simulink model "foptdModel_21a"  (Simulink 10.3)
settings: Solver=FixedStepAuto  StartTime=0.0  StopTime=toutReal(end)-0.3  FixedStep=0.3  RelTol=1e-3
values from neighbouring files (symbols this model uses):
  deltap = [10.95 6 7.8 19.65 17.55 2.85 17.7]    [SimulinkFOPTD-DESKTOP-H1.m]    (also in SimulinkFOPTD.m)
  du = 0.5    [SimulinkFOPTD-DESKTOP-H1.m]    (also in SimulinkFOPTD.m)
  i = input("Wybierz numer skoku (1-7): ")    [SimulinkFOPTD-DESKTOP-H1.m]    (also in SimulinkFOPTD.m)
  taup = [60.75 42.3 39.6 41.85 39.15 20.25 30.6]    [SimulinkFOPTD-DESKTOP-H1.m]    (also in SimulinkFOPTD.m)
  y0 = [59.8 48.9 42.1 37.4 34 31.6 29.7]    [SimulinkFOPTD-DESKTOP-H1.m]    (also in SimulinkFOPTD.m)
undefined symbols (not defined in the file or in its folder): K
settings Model: Creator=danie  LastModifiedBy=hkacp
settings SolverCC: AlgebraicLoopSolver=Auto
settings DataIOCC: SaveFormat=Dataset  SignalLoggingSaveFormat=Dataset  ReturnWorkspaceOutputs=on
settings OptimizationCC: ExpressionDepthLimit=128  LifeSpan=auto
settings DebuggingCC: UnderspecifiedInitializationDetection=Simplified  MergeDetectMultiDrivingBlocksExec=error  FcnCallInpInsideContextMsg=error  StateNameClashWarn=none  SFUnexpectedBacktrackingDiag=error  SFNoUnconditionalDefaultTransitionDiag=error  SFExecutionAtInitializationDiag=warning  SFMachineParentedDataDiag=error  ArithmeticOperatorsInVariantConditions=error
settings HardwareCC: ProdBitPerPointer=64  ProdBitPerSizeT=64  ProdBitPerPtrDiffT=64  ProdLargestAtomicFloat=Float  ProdIntDivRoundTo=Zero  ProdEndianess=LittleEndian  ProdWordSize=64  ProdHWDeviceType=Intel->x86-64 (Windows64)
settings ModelReferenceCC: PropagateSignalLabelsOutOfModel=on
settings SFSimCC: SimUseLocalCustomCode=on  CustomCodeUndefinedFunction=FilterOut
settings RTWCC: RTWUseLocalCustomCode=on
settings CodeAppCC: StateflowObjectComments=off
settings GRTTargetCC: TargetLangStandard=C99 (ISO)  CombineOutputUpdateFcns=on  GRTInterface=off
settings ConfigComp: CovMetricSettings=dwe  CovSaveCumulativeToWorkspaceVar=off  CovSaveSingleToWorkspaceVar=off  CovExternalEMLEnable=on

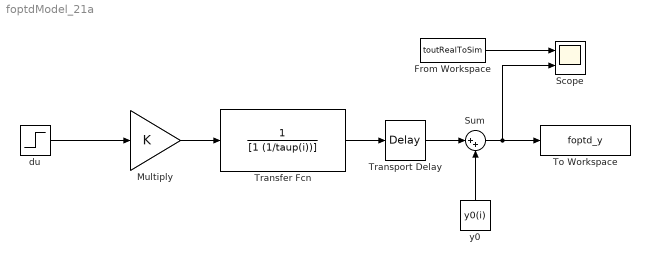
== system foptdModel_21a ==
  From Workspace : FromWorkspace  VariableName=toutRealToSim
  Multiply : Gain  Gain=K
  Scope : Scope  NumInputPorts=2
  Sum : Sum  Inputs=|++
  To Workspace : ToWorkspace  VariableName=foptd_y  SampleTime=-1
  Transfer Fcn : TransferFcn  Denominator=[1 (1/taup(i))]
  Transport Delay : TransportDelay  DelayTime=deltap(i)
  du : Step  Time=0  After=du  SampleTime=0
  y0 : Constant  Value=y0(i)
  wires:
  du/1 -> Multiply/1
  Multiply/1 -> Transfer Fcn/1
  Transfer Fcn/1 -> Transport Delay/1
  Transport Delay/1 -> Sum/1
  y0/1 -> Sum/2
  Sum/1 -> Scope/2, To Workspace/1
  From Workspace/1 -> Scope/1
